simulink model "Two_PSK"  (R2013a)
settings: Solver=ode45  StartTime=0.0  StopTime=10.0  RelTol=1e-3
libraries: dsparch4 x1, commrandsrc2 x1, commsrccod2 x1, commutil2 x1
settings Model: Creator=sliencer  LastModifiedBy=sliencer

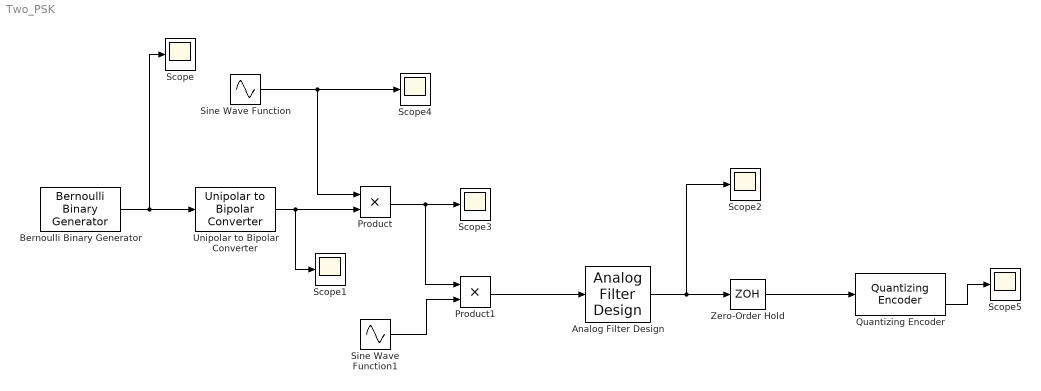
== system Two_PSK ==
  Analog Filter Design : dsparch4/Analog Filter Design  method=Butterworth  filttype=Lowpass  N=8  Wlo=10*pi  Whi=80  Rp=2  Rs=40
  Bernoulli Binary Generator : commrandsrc2/Bernoulli Binary Generator  P=0.5  seed=61  Ts=1  frameBased=off  sampPerFrame=1  orient=off  outDataType=double
  Product : Product
  Product1 : Product
  Quantizing Encoder : commsrccod2/Quantizing Encoder  partition=[0]  codebook=[0 1]  idxDType=double
  Scope{,1..5} (6 alike) : Scope
      Scope2 settings: SaveName=ScopeData2
      Scope3 settings: SaveName=ScopeData3
      Scope4 settings: SaveName=ScopeData4
      Scope5 settings: SaveName=ScopeData5
  Sine Wave Function : Sin  Frequency=10*pi  SampleTime=0
  Sine Wave Function1 : Sin  Frequency=10*pi  SampleTime=0
  Unipolar to Bipolar Converter : commutil2/Unipolar to Bipolar Converter  M=2  polarity=Positive  dataType=Same as input
  Zero-Order Hold : ZeroOrderHold
  wires:
  Bernoulli Binary Generator/1 -> Scope/1, Unipolar to Bipolar Converter/1
  Sine Wave Function/1 -> Scope4/1, Product/1
  Unipolar to Bipolar Converter/1 -> Scope1/1, Product/2
  Product/1 -> Scope3/1, Product1/1
  Sine Wave Function1/1 -> Product1/2
  Zero-Order Hold/1 -> Quantizing Encoder/1
  Analog Filter Design/1 -> Scope2/1, Zero-Order Hold/1
  Product1/1 -> Analog Filter Design/1
  Quantizing Encoder/2 -> Scope5/1
